simulink model "DCspeedpos"  (R2017b)
settings: Solver=VariableStepAuto  StartTime=0.0  StopTime=inf  RelTol=1e-3
libraries: simulink x1, vrlib x1
settings Model: Creator=angel  LastModifiedBy=angel

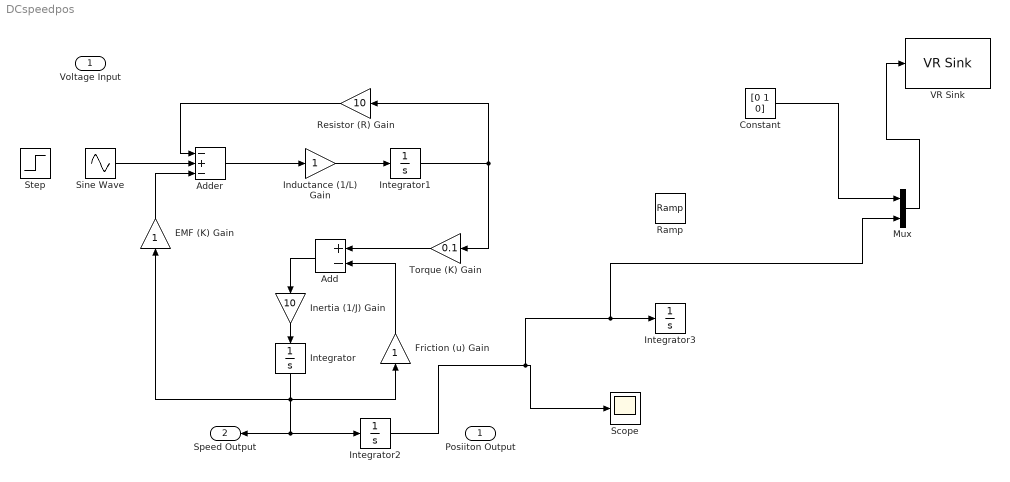
== system DCspeedpos ==
  "Voltage Input " : Inport
  Add : Sum  Inputs=+-
  Adder : Sum  Inputs=-+-
  Constant : Constant  Value=[0 1 0]
  EMF (K) Gain : Gain
  Friction (u) Gain : Gain
  Inductance (1/L) Gain : Gain
  Inertia (1/J) Gain : Gain  Gain=10
  Integrator{,1..3} (4 alike) : Integrator
  Mux : Mux  Inputs=2
  Ramp : simulink/Sources/Ramp  slope=3  start=0  X0=0
  Resistor (R) Gain : Gain  Gain=10
  Scope : Scope
  Sine Wave : Sin  Amplitude=200  Frequency=0.5  SampleTime=0
  Step : Step  SampleTime=0
  Torque (K) Gain : Gain  Gain=0.1
  VR Sink : vrlib/VR Sink  InstantiateOnLoad=on  SampleTime=0.1  ViewEnable=on  RemoteChange=off  RemoteView=off  FieldsWritten=Joint.rotation.4.1.1.double  WorldFileName=MLP\Angel_motor.wrl  AutoView=off  VideoDimensions=[]  AllowVariableSize=off
      settings: SourceProductBaseCode=VR
  Posiiton Output : Outport
  Speed Output : Outport  Port=2
  wires:
  Adder/1 -> Inductance (1/L) Gain/1
  Inductance (1/L) Gain/1 -> Integrator1/1
  Integrator1/1 -> Torque (K) Gain/1, Resistor (R) Gain/1
  Resistor (R) Gain/1 -> Adder/1
  Torque (K) Gain/1 -> Add/1
  Friction (u) Gain/1 -> Add/2
  Add/1 -> Inertia (1/J) Gain/1
  Inertia (1/J) Gain/1 -> Integrator/1
  EMF (K) Gain/1 -> Adder/3
  Constant/1 -> Mux/1
  Mux/1 -> VR Sink/1
  Integrator/1 -> Integrator2/1, Speed Output/1, EMF (K) Gain/1, Friction (u) Gain/1
  Integrator2/1 -> Mux/2, Integrator3/1, Scope/1
  Sine Wave/1 -> Adder/2
